simulink model "Control"  (Simulink 7.9)
settings: Solver=FixedStepDiscrete  StartTime=0.0  StopTime=inf  FixedStep=1/20  RelTol=1e-3
libraries: xpcseriallib x8, dspnetwork x7, simulink x5, instrumentlib x2, aerolibanimutils x2
settings Model: Creator=rgordon  LastModifiedBy=JLEE
settings OptimizationCC: ExpressionDepthLimit=128  OptimizeModelRefInitCode=on  LifeSpan=Inf
settings DebuggingCC: MultiTaskDSMMsg=warning  MultiTaskCondExecSysMsg=none  StrictBusMsg=None
settings RTWCC: SystemTargetFile=ert.tlc  TemplateMakefile=ert_default_tmf  Description=Embedded Coder  ProcessScript=ert_make_rtw_hook  IncludeERTFirstTime=on
settings CodeAppCC: IgnoreCustomStorageClasses=off  CustomSymbolStrType=$N$R$M_T
settings ERTTargetCC: CodeReplacementLibrary=ANSI_C  MultiwordLength=2048  GenerateSampleERTMain=on  SupportNonInlinedSFcns=on  ERTCustomFileTemplate=example_file_process.tlc  ConvertIfToSwitch=off  SuppressUnreachableDefaultCases=off

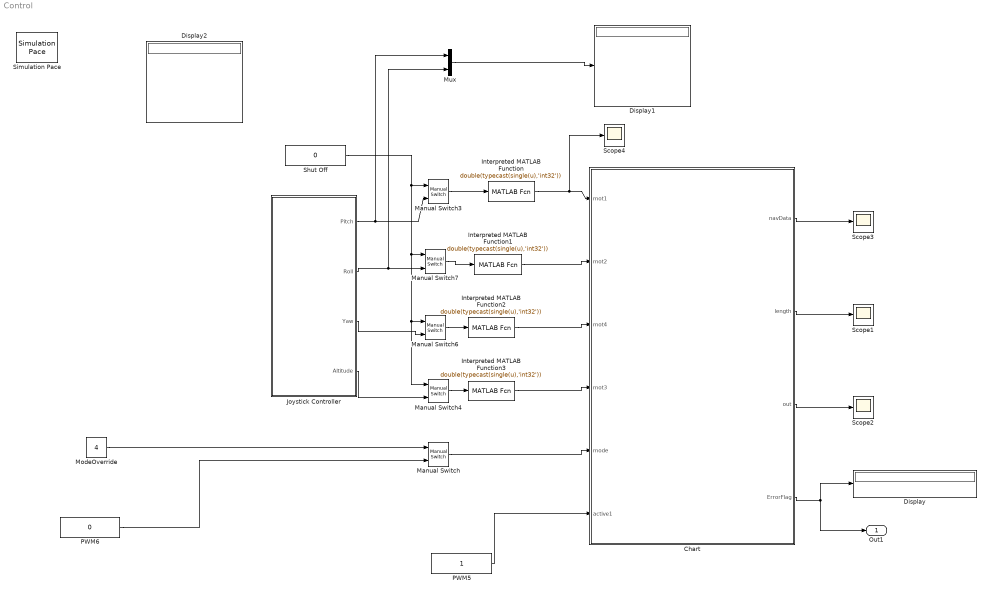
== system Control ==
  Chart : Stateflow chart  TreatAsAtomicUnit=on
  Display : Display
  Display1 : Display
  Display2 : Display
  Interpreted MATLAB Function{,1..3} (4 alike) : MATLABFcn  MATLABFcn=double(typecast(single(u),'int32'))  OutputSignalType=real  Output1D=off
  Joystick Controller : Subsystem
  Manual Switch : simulink/Signal Routing/Manual Switch  sw=1  action=0  varsize=off
  Manual Switch3 : simulink/Signal Routing/Manual Switch  sw=0  action=0  varsize=off
  Manual Switch4 : simulink/Signal Routing/Manual Switch  sw=1  action=0  varsize=off
  Manual Switch6 : simulink/Signal Routing/Manual Switch  sw=0  action=0  varsize=off
  Manual Switch7 : simulink/Signal Routing/Manual Switch  sw=0  action=0  varsize=off
  ModeOverride : Constant  Value=4
  Mux : Mux  Inputs=2
  PWM5 : Constant
  PWM6 : Constant  Value=0
  Scope{1..4} (4 alike) : Scope
      Scope2 settings: TimeRange=10  YMin=0.95  YMax=1.05  SaveName=ScopeData2
      Scope3 settings: SaveName=ScopeData3
      Scope4 settings: YMin=-1.08549e+09  YMax=-1.08549e+09
  Shut Off : Constant  Value=0
  Simulation Pace : aerolibanimutils/Simulation Pace  SimulationPace=1  SleepMode=MATLAB Thread  OutputPaceError=off  SampleTime=1/20
      settings: AttributesFormatString=%<SimulationPace> sec/sec
  Out1 : Outport
  wires:
  Chart/2(length) -> Scope1/1
  Chart/3(out) -> Scope2/1
  Chart/1(navData) -> Scope3/1
  Chart/4(ErrorFlag) -> Display/1, Out1/1
  Interpreted MATLAB Function/1 -> Scope4/1, Chart/1(mot1)
  Interpreted MATLAB Function1/1 -> Chart/2(mot2)
  Interpreted MATLAB Function3/1 -> Chart/4(mot3)
  Interpreted MATLAB Function2/1 -> Chart/3(mot4)
  PWM5/1 -> Chart/6(active1)
  ModeOverride/1 -> Manual Switch/1
  PWM6/1 -> Manual Switch/2
  Manual Switch/1 -> Chart/5(mode)
  Shut Off/1 -> Manual Switch3/1, Manual Switch4/1, Manual Switch6/1, Manual Switch7/1
  Manual Switch3/1 -> Interpreted MATLAB Function/1
  Manual Switch4/1 -> Interpreted MATLAB Function3/1
  Manual Switch6/1 -> Interpreted MATLAB Function2/1
  Manual Switch7/1 -> Interpreted MATLAB Function1/1
  Mux/1 -> Display1/1
  Joystick Controller/4(Altitude) -> Manual Switch4/2
  Joystick Controller/3(Yaw) -> Manual Switch6/2
  Joystick Controller/2(Roll) -> Manual Switch7/2, Mux/2
  Joystick Controller/1(Pitch) -> Manual Switch3/2, Mux/1

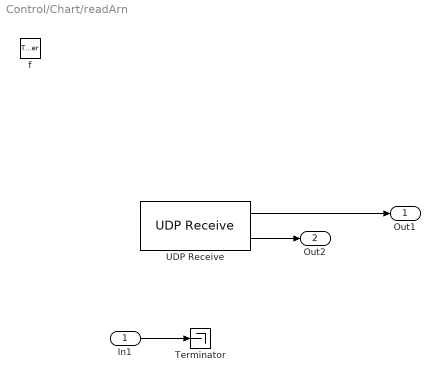
== system Control/Chart/readArn ==
  In1 : Inport
  f : TriggerPort  TriggerType=function-call
      settings: CopyFcn=Stateflow.SLINSF.SimulinkMan.removeBlockPreDeleteFcn  PreDeleteFcn=Stateflow.SLINSF.SimulinkMan.unsafePredeleteFcn
  Terminator : Terminator
  UDP Receive : instrumentlib/UDP Receive  Host=192.168.1.1  Port=5554  LocalPort=5554  DataSize="[292    1]"  EnableBlockingMode=off  Timeout=10  SampleTime=-1  DataType=uint8  ByteOrder=LittleEndian
  Out1 : Outport
  Out2 : Outport  Port=2
  wires:
  In1/1 -> Terminator/1
  UDP Receive/1 -> Out1/1
  UDP Receive/2 -> Out2/1

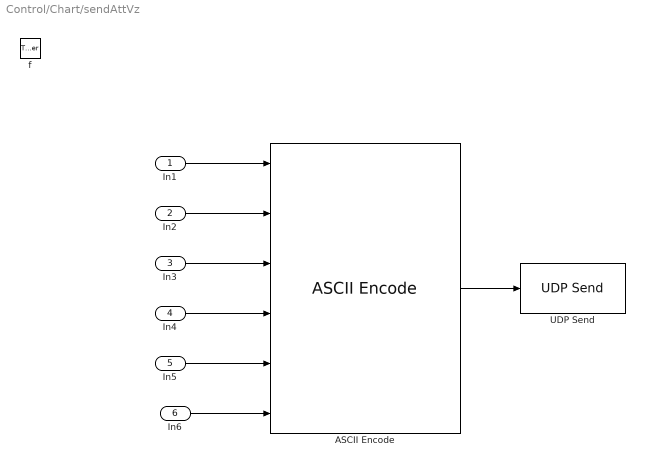
== system Control/Chart/sendAttVz ==
  In1 : Inport
  In2 : Inport  Port=2
  In3 : Inport  Port=3
  In4 : Inport  Port=4
  In5 : Inport  Port=5
  In6 : Inport  Port=6
  f : TriggerPort  TriggerType=function-call
      settings: CopyFcn=Stateflow.SLINSF.SimulinkMan.removeBlockPreDeleteFcn  PreDeleteFcn=Stateflow.SLINSF.SimulinkMan.unsafePredeleteFcn
  "ASCII Encode " : xpcseriallib/ASCII Encode   format=AT*PCMD=%d,%d,%d,%d,%d,%d\r  nvars=6  maxlength=128  vartypes={ 'double' }
  UDP Send : dspnetwork/UDP Send  remoteURL='192.168.1.1'  remotePort=5556  localURL='0.0.0.0'  localPortSource=Specify via dialog  localPort=5556  sampletime=-1  separateLengthPort=0
  wires:
  "ASCII Encode "/1 -> UDP Send/1
  In1/1 -> "ASCII Encode "/1
  In2/1 -> "ASCII Encode "/2
  In3/1 -> "ASCII Encode "/3
  In4/1 -> "ASCII Encode "/4
  In5/1 -> "ASCII Encode "/5
  In6/1 -> "ASCII Encode "/6

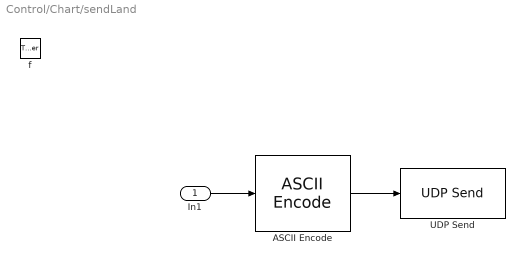
== system Control/Chart/sendLand ==
  In1 : Inport
  f : TriggerPort  TriggerType=function-call
      settings: CopyFcn=Stateflow.SLINSF.SimulinkMan.removeBlockPreDeleteFcn  PreDeleteFcn=Stateflow.SLINSF.SimulinkMan.unsafePredeleteFcn
  "ASCII Encode " : xpcseriallib/ASCII Encode   format=AT*REF=%d,290717696\r  nvars=1  maxlength=128  vartypes={ 'double' }
  UDP Send : dspnetwork/UDP Send  remoteURL='192.168.1.1'  remotePort=5556  localURL='0.0.0.0'  localPortSource=Specify via dialog  localPort=5556  sampletime=-1  separateLengthPort=0
  wires:
  "ASCII Encode "/1 -> UDP Send/1
  In1/1 -> "ASCII Encode "/1

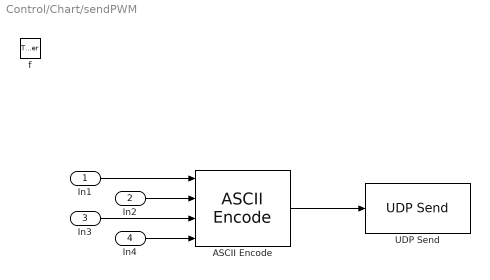
== system Control/Chart/sendPWM ==
  In1 : Inport
  In2 : Inport  Port=2
  In3 : Inport  Port=3
  In4 : Inport  Port=4
  f : TriggerPort  TriggerType=function-call
      settings: CopyFcn=Stateflow.SLINSF.SimulinkMan.removeBlockPreDeleteFcn  PreDeleteFcn=Stateflow.SLINSF.SimulinkMan.unsafePredeleteFcn
  "ASCII Encode " : xpcseriallib/ASCII Encode   format=AT*PWM=1,%d,%d,%d,%d\r  nvars=4  maxlength=128  vartypes={ 'double' }
  UDP Send : dspnetwork/UDP Send  remoteURL='192.168.1.1'  remotePort=5556  localURL='0.0.0.0'  localPortSource=Specify via dialog  localPort=5556  sampletime=-1  separateLengthPort=0
  wires:
  "ASCII Encode "/1 -> UDP Send/1
  In1/1 -> "ASCII Encode "/1
  In2/1 -> "ASCII Encode "/2
  In3/1 -> "ASCII Encode "/3
  In4/1 -> "ASCII Encode "/4

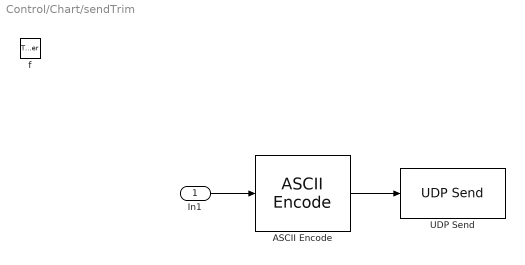
== system Control/Chart/sendTrim ==
  In1 : Inport
  f : TriggerPort  TriggerType=function-call
      settings: CopyFcn=Stateflow.SLINSF.SimulinkMan.removeBlockPreDeleteFcn  PreDeleteFcn=Stateflow.SLINSF.SimulinkMan.unsafePredeleteFcn
  "ASCII Encode " : xpcseriallib/ASCII Encode   format=AT*FTRIM=%d,\r  nvars=1  maxlength=128  vartypes={ 'double' }
  UDP Send : dspnetwork/UDP Send  remoteURL='192.168.1.1'  remotePort=5556  localURL='0.0.0.0'  localPortSource=Specify via dialog  localPort=5556  sampletime=-1  separateLengthPort=0
  wires:
  "ASCII Encode "/1 -> UDP Send/1
  In1/1 -> "ASCII Encode "/1

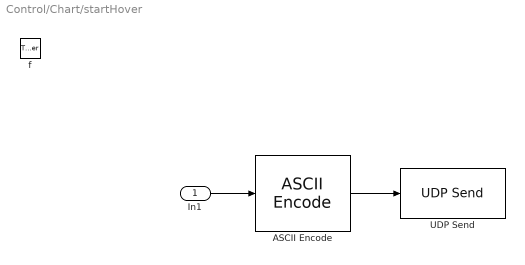
== system Control/Chart/startHover ==
  In1 : Inport
  f : TriggerPort  TriggerType=function-call
      settings: CopyFcn=Stateflow.SLINSF.SimulinkMan.removeBlockPreDeleteFcn  PreDeleteFcn=Stateflow.SLINSF.SimulinkMan.unsafePredeleteFcn
  "ASCII Encode " : xpcseriallib/ASCII Encode   format=AT*REF=%d,290718208\r  nvars=1  maxlength=128  vartypes={ 'double' }
  UDP Send : dspnetwork/UDP Send  remoteURL='192.168.1.1'  remotePort=5556  localURL='0.0.0.0'  localPortSource=Specify via dialog  localPort=5556  sampletime=-1  separateLengthPort=0
  wires:
  "ASCII Encode "/1 -> UDP Send/1
  In1/1 -> "ASCII Encode "/1

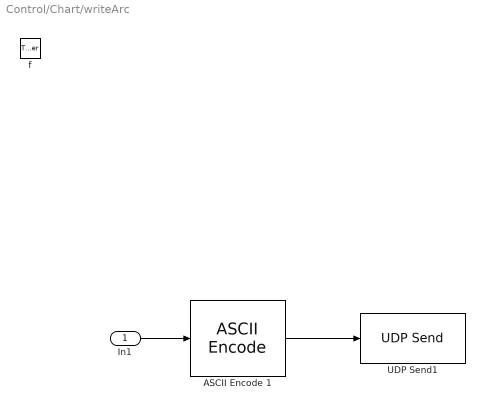
== system Control/Chart/writeArc ==
  In1 : Inport
  f : TriggerPort  TriggerType=function-call
      settings: CopyFcn=Stateflow.SLINSF.SimulinkMan.removeBlockPreDeleteFcn  PreDeleteFcn=Stateflow.SLINSF.SimulinkMan.unsafePredeleteFcn
  ASCII Encode 1 : xpcseriallib/ASCII Encode   format='AT*COMWDG=,%d,\r  nvars=1  maxlength=128  vartypes={ 'double' }
  UDP Send1 : dspnetwork/UDP Send  remoteURL='192.168.1.1'  remotePort=5556  localURL='0.0.0.0'  localPortSource=Specify via dialog  localPort=5556  sampletime=-1  separateLengthPort=0
  wires:
  ASCII Encode 1/1 -> UDP Send1/1
  In1/1 -> ASCII Encode 1/1

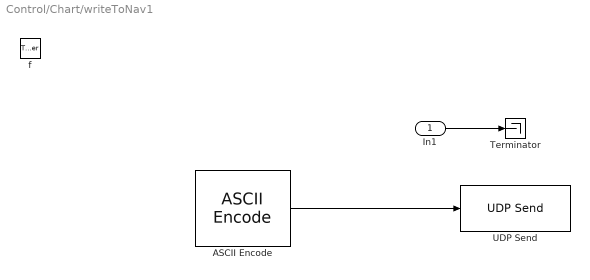
== system Control/Chart/writeToNav1 ==
  In1 : Inport
  f : TriggerPort  TriggerType=function-call
      settings: CopyFcn=Stateflow.SLINSF.SimulinkMan.removeBlockPreDeleteFcn  PreDeleteFcn=Stateflow.SLINSF.SimulinkMan.unsafePredeleteFcn
  "ASCII Encode " : xpcseriallib/ASCII Encode   format=1  nvars=0  maxlength=128  vartypes={ 'double' }
  Terminator : Terminator
  UDP Send : instrumentlib/UDP Send  Host=192.168.1.1  Port=5554  LocalPort=5554  EnableBlockingMode=off  ByteOrder=BigEndian
  wires:
  "ASCII Encode "/1 -> UDP Send/1
  In1/1 -> Terminator/1

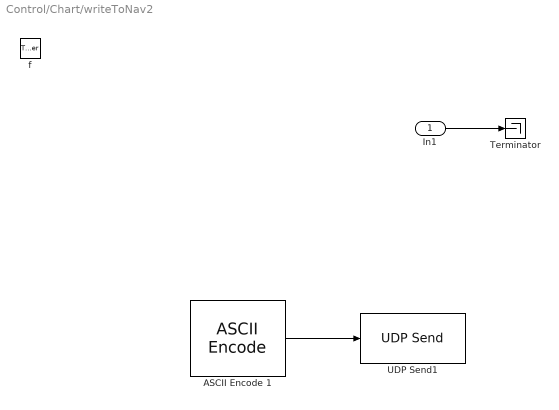
== system Control/Chart/writeToNav2 ==
  In1 : Inport
  f : TriggerPort  TriggerType=function-call
      settings: CopyFcn=Stateflow.SLINSF.SimulinkMan.removeBlockPreDeleteFcn  PreDeleteFcn=Stateflow.SLINSF.SimulinkMan.unsafePredeleteFcn
  ASCII Encode 1 : xpcseriallib/ASCII Encode   format="AT*CONFIG=2,\\\"general:navdata_demo\\\",\\\"TRUE\\\"\\r"  nvars=0  maxlength=128  vartypes={ 'double' }
  Terminator : Terminator
  UDP Send1 : dspnetwork/UDP Send  remoteURL='192.168.1.1'  remotePort=5556  localURL='0.0.0.0'  localPortSource=Specify via dialog  localPort=5556  sampletime=-1  separateLengthPort=0
  wires:
  In1/1 -> Terminator/1
  ASCII Encode 1/1 -> UDP Send1/1

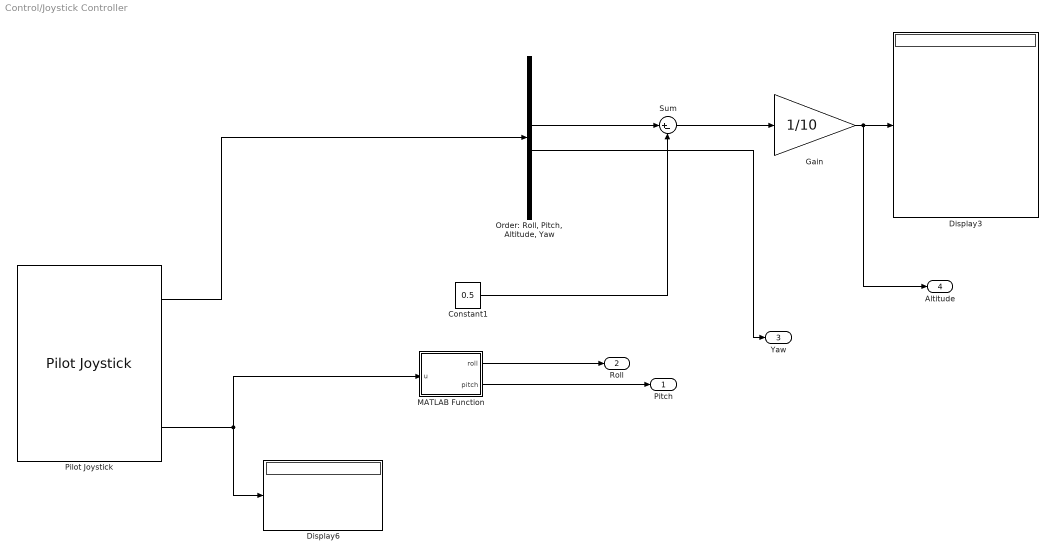
== system Control/Joystick Controller ==
  Constant1 : Constant  Value=0.5
  Display3 : Display
  Display6 : Display
  Gain : Gain  Gain=1/10
  MATLAB Function : MATLAB Function  TreatAsAtomicUnit=on
  "Order: Roll, Pitch, Altitude, Yaw" : Demux  Outputs=6
  Pilot Joystick : aerolibanimutils/Pilot Joystick  JoystickID=Joystick1  OutputConfiguration=AllOutputs  SampleTime=-1
  Sum : Sum  Inputs=|+-
  Pitch : Outport
  Roll : Outport  Port=2
  Yaw : Outport  Port=3
  Altitude : Outport  Port=4
  wires:
  Pilot Joystick/1 -> "Order: Roll, Pitch, Altitude, Yaw"/1
  Pilot Joystick/3 -> Display6/1, MATLAB Function/1(u)
  "Order: Roll, Pitch, Altitude, Yaw"/3 -> Sum/1
  Constant1/1 -> Sum/2
  Sum/1 -> Gain/1
  MATLAB Function/1(roll) -> Roll/1
  MATLAB Function/2(pitch) -> Pitch/1
  Gain/1 -> Display3/1, Altitude/1
  "Order: Roll, Pitch, Altitude, Yaw"/4 -> Yaw/1

== stateflow chart Chart ==
  state RunMotor2
    entry:ErrorFlag = 0;
    during: sendAttVz(mot1,mot2,mot3,mot4,i,active1)
  state sendPWM(In1,In2,In3,In4) [function]
  state RunMotor1
    entry:ErrorFlag = 0;
    during: sendPWM(mot1,mot2,mot3,mot4)
  state MotorCmdError
    entry:ErrorFlag = 1;
  state ModeSelector
  state RunMotor3
    entry:ErrorFlag = 0;
    during: sendTrim(i)
  state RunMotor5
    entry:ErrorFlag = 0;
    during: startHover(1)
  state startHover(In1) [function]
  state sendTrim(In1) [function]
  state wait
  state RunMotor4
    entry:ErrorFlag = 0;
    during: sendAttVz(i,active1,mot1,mot2,mot3,mot4)
  state RunMotor6
    entry:ErrorFlag = 0;
    during: sendLand(i)
  state RunNav
    state writeToArc
      entry:writeArc(i)
    state writeToArc1
      entry:[navData,length] = readArn(1)
    (default) -> writeToArc
    writeToArc -> writeToArc1 : after(0.5,sec)
        | {out=i;
        | i=i+1;}
    writeToArc1 -> writeToArc : after(0.5,sec)
  state writeToNav1(In1) [function]
  state writeToNav2(In1) [function]
  state sendLand(In1) [function]
  state writeArc(In1) [function]
  state sendAttVz(In1,In2,In3,In4,In5,In6) [function]
  state [Out1,Out2] = readArn(In1) [function]
  (default) -> (junction 24)
  RunMotor2 -> ModeSelector : [mode~=3]
  ModeSelector -> RunMotor2 [order 3] : [mode == 3]
  (junction 24) -> ModeSelector : {i = 1}
  RunMotor1 -> MotorCmdError [order 2] : [mot1>255 || mot2>255 || mot3>255 || mot4>255]
  RunMotor1 -> ModeSelector [order 1] : [mode~=1]
  RunMotor3 -> ModeSelector [order 1] : [mode~=4]
  RunMotor3 -> RunMotor5 [order 2] : after(5,sec)
      | {i=i+1;}
  ModeSelector -> RunMotor3 [order 4] : [mode == 4]
      | {i=i+1;}
  MotorCmdError -> RunMotor1 : [mot1<256 && mot2<256 && mot3<256 && mot4<256
      | ]
  ModeSelector -> RunMotor1 [order 1] : [mode==1]
  RunMotor6 -> ModeSelector : after(1,sec)
  RunNav -> ModeSelector : [mode~=2]
  ModeSelector -> wait [order 2] : [mode==2]
      | {writeToNav1(1);
      |  i = 1000;}
  RunMotor5 -> RunMotor4 : after(1,sec)
      | {i=i+1;}
  wait -> RunNav : after(0.5,sec)
      | {writeToNav2(1);}
  RunMotor4 -> RunMotor6 [order 1] : [mode~=4]
      | {i=i+1;}
  RunMotor4 -> RunMotor4 [order 2] : after(0.5,sec)
      | {i=i+1;}
  data: In1 function_input double; In2 function_input double; In3 function_input double; In4 function_input double; In1 function_input double; In1 function_input double; In1 function_input double; In1 function_input double; In1 function_input double; In1 function_input double; In1 function_input double; In2 function_input double; In3 function_input double; In4 function_input double; In5 function_input double; In6 function_input double; In1 function_input double; Out1 function_output double; Out2 function_output double; mot1 input double; mot2 input double; mot4 input double; mot3 input double; mode input double; i local double; navData output uint8 size=[292,1]; length output double; out output double; ErrorFlag output double; active1 input double

== matlab function Joystick Controller/MATLAB Function ==
  data: u input double; roll output double; pitch output double
function [roll,pitch] = fcn(u)
%#codegen

if u == 0
    roll  = 0;
    pitch = -0.2;
%     yaw   = 
elseif u == 180
    roll  = 0;
    pitch = 0.2;
%     yaw   = 
    
elseif u == 90
    roll  = 0.2;
    pitch = 0;
%     yaw   = 
    
elseif u == 270
    roll  = -0.2;
    pitch = 0;
%     yaw   = 
else
    
    roll  = 0;
    pitch = 0;
%     yaw   = 0;
    
end
